simulink model "modele_simulink"  (R2025b)
settings: Solver=VariableStepAuto  StartTime=0.0  StopTime=10.0  RelTol=1e-3
values from neighbouring files (symbols this model uses):
  fD = 2*v_target/(c/f0)    (= 3200)    [test.m]
  Fs = 5e9    (= 5000000000)    [test.m]
undefined symbols (not defined in the file or in its folder): tau_samples
libraries: dspsigops x1
settings Model: Creator=Antoine  LastModifiedBy=Antoine

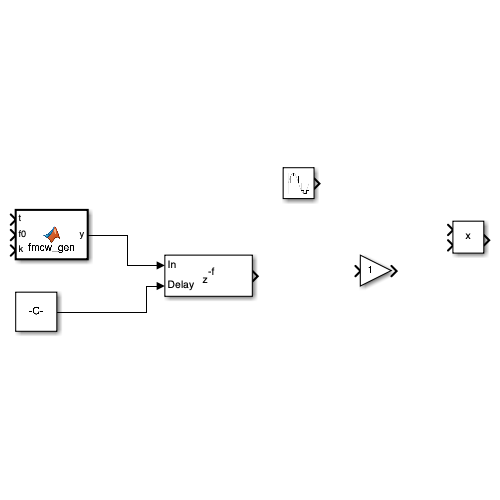
[thumbnail: Simulink's stored preview of the top-level diagram]
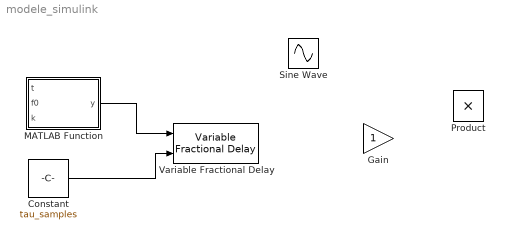
== system modele_simulink ==
  Constant : Constant  Value=tau_samples
  Gain : Gain
  MATLAB Function : MATLAB Function  TreatAsAtomicUnit=on
  Product : Product
  Sine Wave : Sin  Frequency=fD  SampleTime=1/Fs
  Variable Fractional Delay : dspsigops/Variable Fractional Delay  mode=OBSOLETE  modeActive=Linear  L=4  FarrowL=4  R=10  alpha=1  dmax=100  InputProcessing=Columns as channels (frame based)  ic=0  noDFT=off  fallbackFIR=Clip to the minimum value necessary for centered kernel  fallbackFarrow=Clip to the minimum value necessary for centered kernel  roundingMode=Zero  overflowMode=off
  wires:
  MATLAB Function/1(y) -> Variable Fractional Delay/1
  Constant/1 -> Variable Fractional Delay/2

== matlab function modele_simulink/MATLAB Function ==
  data: t input; y output; f0 input; k input
function y = fmcw_gen(t, f0, k)
    phase = 2*pi*(f0*t + 0.5*k*t*t);
    y = exp(1j*phase);
end
